simulink model "AnInductorExample"  (R2020b)
settings: Solver=VariableStepAuto  StartTime=0.0  StopTime=1  RelTol=1e-3
libraries: powerlib x8
settings Model: Creator=admin_user  LastModifiedBy=admin_user

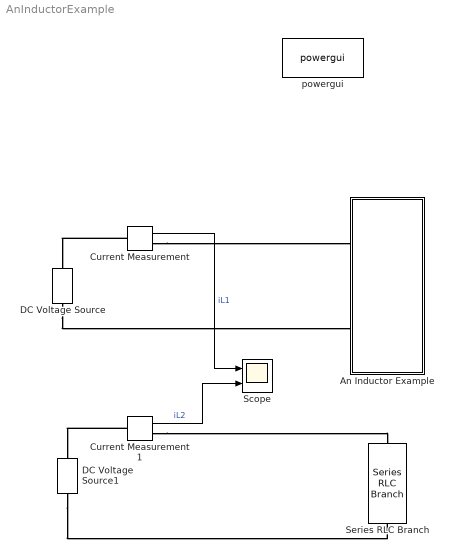
== system AnInductorExample ==
  An Inductor Example : Subsystem  mask{Ts=1/(10*1e3), L=2}
  Current Measurement : powerlib/Measurements/Current Measurement  PhasorSimulation=off  OutputType=Complex  PSBequivalent=0
  Current Measurement1 : powerlib/Measurements/Current Measurement  PhasorSimulation=off  OutputType=Complex  PSBequivalent=0
  DC Voltage Source : powerlib/Electrical Sources/DC Voltage Source  Amplitude=1  Measurements=None
  DC Voltage Source1 : powerlib/Electrical Sources/DC Voltage Source  Amplitude=1  Measurements=None
  Scope : Scope  NumInputPorts=2
  Series RLC Branch : powerlib/Elements/Series RLC Branch  LConnTagsString=__new0  RConnTagsString=__new0  BranchType=L  Resistance=2  Inductance=2  SetiL0=off  InitialCurrent=0  Capacitance=1e-6  Setx0=off  InitialVoltage=0  Measurements=None
  powergui : powerlib/powergui  Priority=1  SimulationMode=Discrete  SampleTime=1/(10*1e3)  frequency=60  Iterations=50  frequencyindice=0  Pbase=100e6  ErrMax=1e-4  UnitsV=kV  UnitsW=MW  buscounter=0  FunctionMessages=off  echomessages=off  EnableUseOfTLC=off  CurrentSourceSwitches=off  DisableSnubberDevices=off  DisableRonSwitches=off  DisableVfSwitches=off  DisplayEquations=off  AutomaticDiscreteSolvers=off  SolverType=Tustin/Backward Euler (TBE)  Interpol=off  ExternalGateDelay=off  methode=off  Ts=100  x0status=blocks  SPID=on  SwTol=0  HookPort=off  NonlinearTolerance=1e-4  nMaxIteration=100  ContinueOnMaxIteration=off  RestoreLinks=warning  ResistiveCurrentMeasurement=off  Frange=[0:2:500]  Ylog=off  Xlog=on  ShowGrid=off  save=off  variable=ZData  structure=0  ZoomFFT=off  StartTime=0.0  cycles=1  DisplayStyle=1  fundamental=60  FreqAxis=off  MaxFrequency=1000  frequencyindicesteady=1  RmsSteady=1  display=off
  wires:
  Current Measurement/1 -> Scope/1  "iL1"
  Current Measurement1/1 -> Scope/2  "iL2"
  connections:
  DC Voltage Source/LConn1 -- An Inductor Example/LConn2
  Current Measurement/LConn1 -- DC Voltage Source/RConn1
  Current Measurement/RConn1 -- An Inductor Example/LConn1
  Current Measurement1/LConn1 -- DC Voltage Source1/RConn1
  DC Voltage Source1/LConn1 -- Series RLC Branch/RConn1
  Current Measurement1/RConn1 -- Series RLC Branch/LConn1

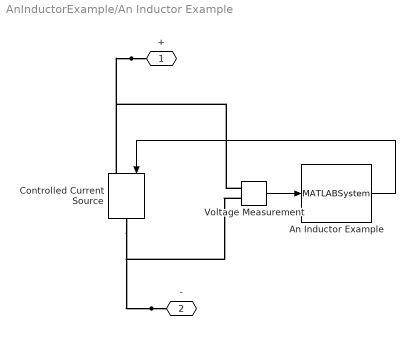
== system AnInductorExample/An Inductor Example ==
  An Inductor Example : MATLABSystem  System=SimplexPS.Class.Inductor  Ts=Ts  Para=L  DeviceType=0  PowerFlow=0  x0=0  DiscreMethod=2  LinearizationTimes=1  DirectFeedthrough=true  VirtualResistor=true  EquiInitial=true  SimulateUsing=Code generation
      mask Type: SimplexPS.Class.Inductor
      mask Display:
      | disp('Inductor');
      | port_label('input',1,'u');
      | port_label('output',1,'y');
  Controlled Current Source : powerlib/Electrical Sources/Controlled Current Source  Initialize=on  Source_Type=AC  Amplitude=0  Phase=0  Frequency=0  Measurements=None
  Voltage Measurement : powerlib/Measurements/Voltage Measurement  PhasorSimulation=off  OutputType=Complex  PSBequivalent=0
  + : PMIOPort  Side=Left
  - : PMIOPort  Port=2  Side=Left
  wires:
  Voltage Measurement/1 -> An Inductor Example/1
  An Inductor Example/1 -> Controlled Current Source/1
  connections:
  -/RConn1 -- Voltage Measurement/LConn2 -- Controlled Current Source/RConn1
  +/RConn1 -- Voltage Measurement/LConn1 -- Controlled Current Source/LConn1
